simulink model "SI_Engine"  (R2020a)
settings: Solver=VariableStepAuto  StartTime=0.0  StopTime=inf  RelTol=1e-3
PostLoadFcn:
  | data1=xlsread('performancemaps','VE');
  | rpm1=data1(1,2:end);
  | map1=data1(2:end,1);
  | ve=data1(2:end,2:end);
  | data2=xlsread('performancemaps','Spark');
  | rpm2=data2(1,2:end);
  | map2=data2(2:end,1);
  | spark=data2(2:end,2:end);
  | data3=xlsread('performancemaps','AFR');
  | rpm3=data3(1,2:end);
  | map3=data3(2:end,1);
  | AFR=data3(2:end,2:end);
settings Model: Creator=sateeshk  LastModifiedBy=sateeshk

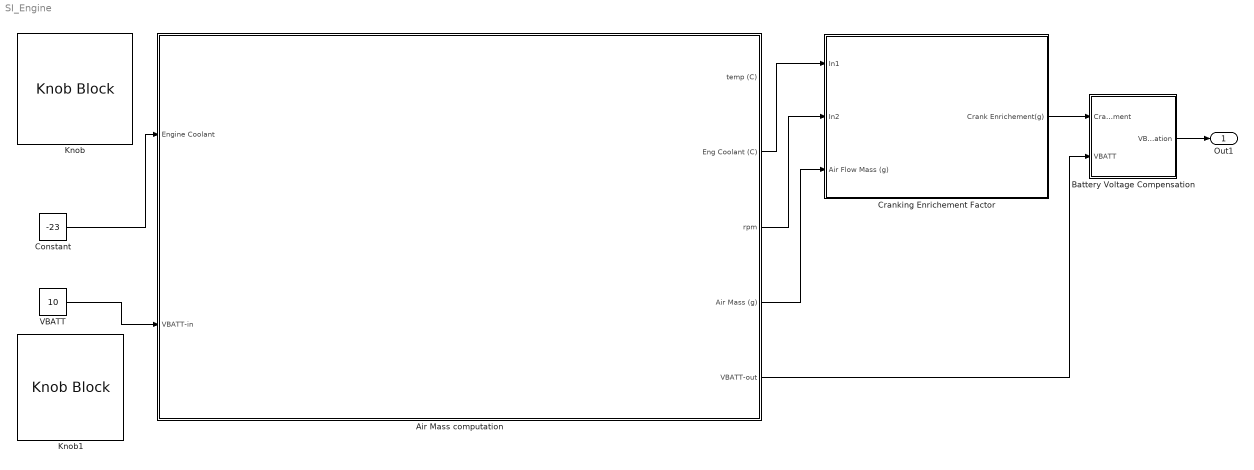
== system SI_Engine ==
  Air Mass computation : Subsystem
  Battery Voltage Compensation : Subsystem
  Constant : Constant  Value=-23
  Cranking Enrichement Factor : Subsystem
  Knob : KnobBlock  ScaleMin=1000  ScaleMax=10000
  Knob1 : KnobBlock  ScaleMin=25  ScaleMax=101
  VBATT : Constant  Value=10
  Out1 : Outport
  wires:
  Constant/1 -> Air Mass computation/1(Engine Coolant)
  Air Mass computation/2(Eng Coolant (C)) -> Cranking Enrichement Factor/1(In1)
  Air Mass computation/3(rpm) -> Cranking Enrichement Factor/2(In2)
  Air Mass computation/4(Air Mass (g)) -> Cranking Enrichement Factor/3(Air Flow Mass (g))
  VBATT/1 -> Air Mass computation/2(VBATT-in)
  Cranking Enrichement Factor/1(Crank Enrichement(g)) -> Battery Voltage Compensation/1(Crank Enrichement)
  Air Mass computation/5(VBATT-out) -> Battery Voltage Compensation/2(VBATT)
  Battery Voltage Compensation/1(VBATT-Compensation) -> Out1/1

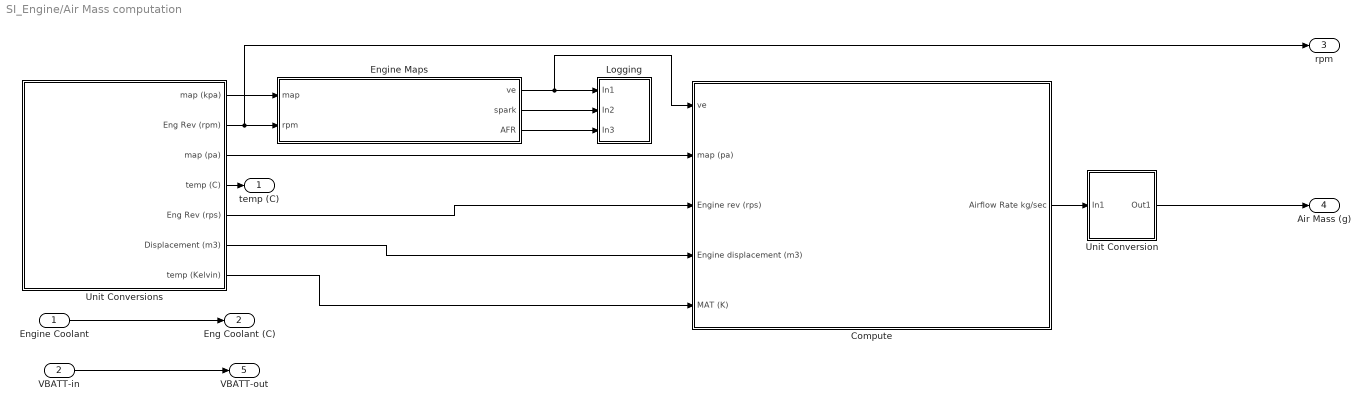
== system SI_Engine/Air Mass computation ==
  Engine Coolant : Inport
  VBATT-in : Inport  Port=2
  Compute : Subsystem
  Engine Maps : Subsystem
  Logging : Subsystem
  Unit Conversion : Subsystem
  Unit Conversions : Subsystem
  temp (C) : Outport
  Eng Coolant (C) : Outport  Port=2
  rpm : Outport  Port=3
  Air Mass (g) : Outport  Port=4
  VBATT-out : Outport  Port=5
  wires:
  Unit Conversion/1(Out1) -> Air Mass (g)/1
  Unit Conversions/2(Eng Rev (rpm)) -> rpm/1, Engine Maps/2(rpm)
  Engine Maps/3(AFR) -> Logging/3(In3)
  Compute/1(Airflow Rate kg/sec) -> Unit Conversion/1(In1)
  Unit Conversions/3(map (pa)) -> Compute/2(map (pa))
  Unit Conversions/6(Displacement (m3)) -> Compute/4(Engine displacement (m3))
  Unit Conversions/1(map (kpa)) -> Engine Maps/1(map)
  Unit Conversions/7(temp (Kelvin)) -> Compute/5(MAT (K))
  Unit Conversions/4(temp (C)) -> temp (C)/1
  Engine Maps/2(spark) -> Logging/2(In2)
  Engine Maps/1(ve) -> Compute/1(ve), Logging/1(In1)
  Unit Conversions/5(Eng Rev (rps)) -> Compute/3(Engine rev (rps))
  Engine Coolant/1 -> Eng Coolant (C)/1
  VBATT-in/1 -> VBATT-out/1

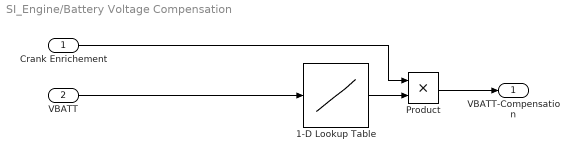
== system SI_Engine/Battery Voltage Compensation ==
  Crank Enrichement : Inport
  VBATT : Inport  Port=2
  1-D Lookup Table : Lookup_n-D  NumberOfTableDimensions=1  BreakpointsForDimension1=[7,10,12,15]  Table=[ 1.3,1.2, 1.0 ,0.9]  InternalRulePriority=Speed  RndMeth=Simplest  InputSameDT=on
  Product : Product
  VBATT-Compensation : Outport
  wires:
  Product/1 -> VBATT-Compensation/1
  VBATT/1 -> 1-D Lookup Table/1
  Crank Enrichement/1 -> Product/1
  1-D Lookup Table/1 -> Product/2

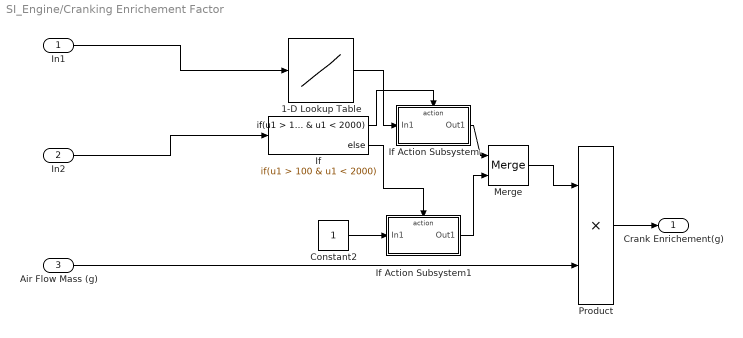
== system SI_Engine/Cranking Enrichement Factor ==
  In1 : Inport
  In2 : Inport  Port=2
  Air Flow Mass (g) : Inport  Port=3
  1-D Lookup Table : Lookup_n-D  NumberOfTableDimensions=1  BreakpointsForDimension1=[-40,-20,-5,15,35,50,70,90]  Table=[1.4,1.25,1.15,1.1,1,1,1,1]  InternalRulePriority=Speed  RndMeth=Simplest  InputSameDT=on
  Constant2 : Constant
  If : If  IfExpression=u1 > 100 & u1 < 2000
  If Action Subsystem : Subsystem  TreatAsAtomicUnit=on
  If Action Subsystem1 : Subsystem  TreatAsAtomicUnit=on
  Merge : Merge
  Product : Product
  Crank Enrichement(g) : Outport
  wires:
  In1/1 -> 1-D Lookup Table/1
  In2/1 -> If/1
  If Action Subsystem/1(Out1) -> Merge/1
  If Action Subsystem1/1(Out1) -> Merge/2
  Constant2/1 -> If Action Subsystem1/1(In1)
  If/1 -> If Action Subsystem/Action
  1-D Lookup Table/1 -> If Action Subsystem/1(In1)
  If/2 -> If Action Subsystem1/Action
  Merge/1 -> Product/1
  Air Flow Mass (g)/1 -> Product/2
  Product/1 -> Crank Enrichement(g)/1

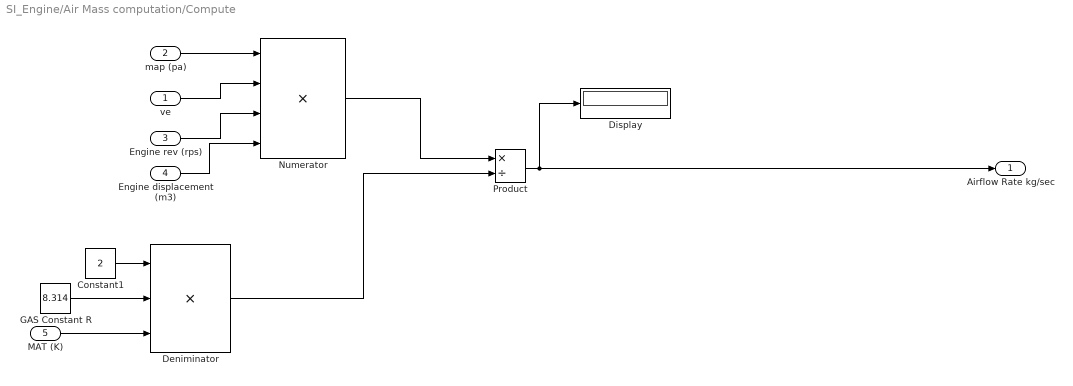
== system SI_Engine/Air Mass computation/Compute ==
  ve : Inport
  map (pa) : Inport  Port=2
  Engine rev (rps) : Inport  Port=3
  Engine displacement (m3) : Inport  Port=4
  MAT (K) : Inport  Port=5
  Constant1 : Constant  Value=2
  Deniminator : Product  Inputs=***
  Display : Display
  GAS Constant R : Constant  Value=8.314
  Numerator : Product  Inputs=****
  Product : Product  Inputs=*/
  Airflow Rate kg/sec : Outport
  wires:
  Constant1/1 -> Deniminator/1
  GAS Constant R/1 -> Deniminator/2
  MAT (K)/1 -> Deniminator/3
  Product/1 -> Display/1, Airflow Rate kg/sec/1
  map (pa)/1 -> Numerator/1
  ve/1 -> Numerator/2
  Engine rev (rps)/1 -> Numerator/3
  Engine displacement (m3)/1 -> Numerator/4
  Numerator/1 -> Product/1
  Deniminator/1 -> Product/2

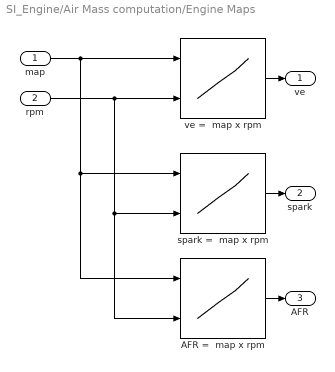
== system SI_Engine/Air Mass computation/Engine Maps ==
  map : Inport
  rpm : Inport  Port=2
  AFR =  map x rpm : Lookup_n-D  BreakpointsForDimension1=map1  BreakpointsForDimension2=rpm1  Table=AFR  InternalRulePriority=Speed  RndMeth=Simplest  InputSameDT=on
  spark =  map x rpm : Lookup_n-D  BreakpointsForDimension1=map1  BreakpointsForDimension2=rpm1  Table=spark  InternalRulePriority=Speed  RndMeth=Simplest  InputSameDT=on
  ve =  map x rpm : Lookup_n-D  BreakpointsForDimension1=map1  BreakpointsForDimension2=rpm1  Table=ve  InternalRulePriority=Speed  RndMeth=Simplest  InputSameDT=on
  ve : Outport
  spark : Outport  Port=2
  AFR : Outport  Port=3
  wires:
  AFR =  map x rpm/1 -> AFR/1
  map/1 -> AFR =  map x rpm/1, spark =  map x rpm/1, ve =  map x rpm/1
  rpm/1 -> AFR =  map x rpm/2, spark =  map x rpm/2, ve =  map x rpm/2
  ve =  map x rpm/1 -> ve/1
  spark =  map x rpm/1 -> spark/1

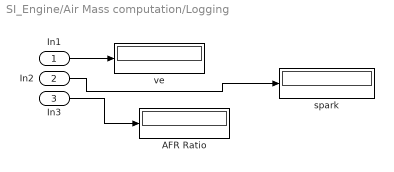
== system SI_Engine/Air Mass computation/Logging ==
  In1 : Inport
  In2 : Inport  Port=2
  In3 : Inport  Port=3
  AFR Ratio : Display
  spark : Display
  ve : Display
  wires:
  In1/1 -> ve/1
  In2/1 -> spark/1
  In3/1 -> AFR Ratio/1

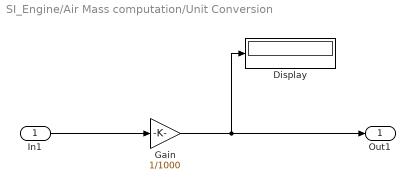
== system SI_Engine/Air Mass computation/Unit Conversion ==
  In1 : Inport
  Display : Display
  Gain : Gain  Gain=1/1000
  Out1 : Outport
  wires:
  In1/1 -> Gain/1
  Gain/1 -> Out1/1, Display/1

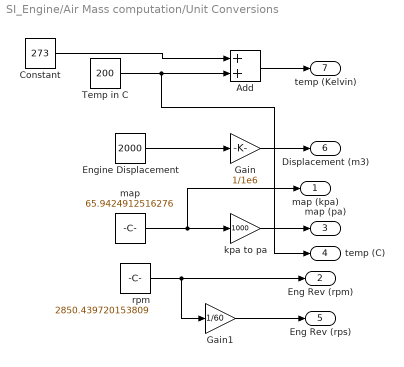
== system SI_Engine/Air Mass computation/Unit Conversions ==
  Add : Sum
  Constant : Constant  Value=273
  Engine Displacement : Constant  Value=2000
  Gain : Gain  Gain=1/1e6
  Gain1 : Gain  Gain=1/60
  Temp in C : Constant  Value=200
  kpa to pa : Gain  Gain=1000
  map : Constant  Value=65.9424912516276
  rpm : Constant  Value=2850.439720153809
  map (kpa) : Outport
  Eng Rev (rpm) : Outport  Port=2
  map (pa) : Outport  Port=3
  temp (C) : Outport  Port=4
  Eng Rev (rps) : Outport  Port=5
  Displacement (m3) : Outport  Port=6
  temp (Kelvin) : Outport  Port=7
  wires:
  rpm/1 -> Gain1/1, Eng Rev (rpm)/1
  Temp in C/1 -> temp (C)/1, Add/2
  Constant/1 -> Add/1
  Engine Displacement/1 -> Gain/1
  map/1 -> map (kpa)/1, kpa to pa/1
  Gain/1 -> Displacement (m3)/1
  kpa to pa/1 -> map (pa)/1
  Add/1 -> temp (Kelvin)/1
  Gain1/1 -> Eng Rev (rps)/1

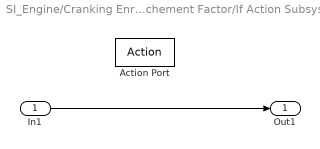
== system SI_Engine/Cranking Enrichement Factor/If Action Subsystem ==
  In1 : Inport
  Action Port : ActionPort  ActionPortLabel=if(u1 > 100 & u1 < 2000)
  Out1 : Outport
  wires:
  In1/1 -> Out1/1

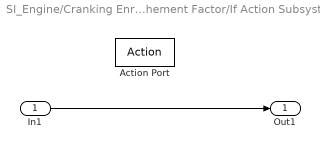
== system SI_Engine/Cranking Enrichement Factor/If Action Subsystem1 ==
  In1 : Inport
  Action Port : ActionPort  ActionPortLabel=else
  Out1 : Outport
  wires:
  In1/1 -> Out1/1
